simulink model "ImpedanceScanAndRecord_v2_for_RTLAB"  (R2020a)
settings: Solver=FixedStepDiscrete  StartTime=0.0  StopTime=30  RelTol=1e-3
InitFcn:
  | Ts = 50e-6;
libraries: dspsigops x16, powerlib x9
settings Model: Creator=anony  LastModifiedBy=anony

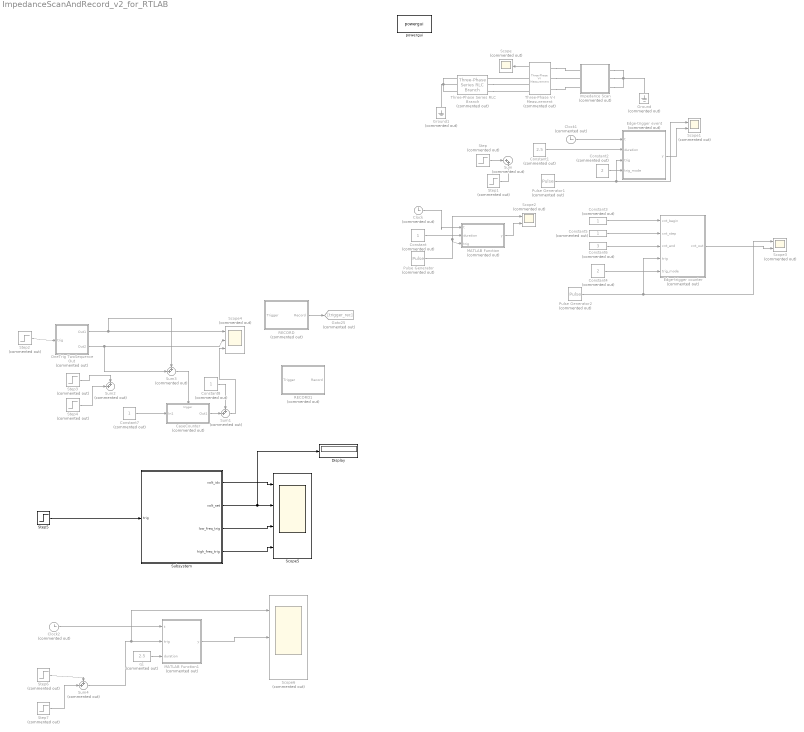
== system ImpedanceScanAndRecord_v2_for_RTLAB ==
  CaseCounter : Subsystem  Commented=on  TreatAsAtomicUnit=on
  Clock : Clock  Commented=on
  Clock1 : Clock  Commented=on
  Clock2 : Clock  Commented=on
  Constant{,3,5,7..8} (5 alike) : Constant  Commented=on
  Constant1 : Constant  Commented=on  Value=2.5
  Constant2 : Constant  Commented=on  Value=2
  Constant4 : Constant  Commented=on  Value=2
  Constant6 : Constant  Commented=on  Value=3
  Display : Display
  Edge-trigger counter : MATLAB Function  Commented=on  TreatAsAtomicUnit=on  SystemSampleTime=50e-6
  Edge-trigger event : MATLAB Function  Commented=on  TreatAsAtomicUnit=on  SystemSampleTime=50e-6
  Goto25 : Goto  Commented=on  GotoTag=trigger_rec
  Ground : powerlib/Elements/Ground  Commented=on  LConnTagsString=a
  Ground1 : powerlib/Elements/Ground  Commented=on  LConnTagsString=a
  Impedance Scan : Subsystem  Commented=on  mask{t_start=1, frequency=1, inject_duration=2, record_duration=1, stable_duration=1, amp_inject=690 * 0.1, t_Ts=Ts}
      mask prompts: t_start "启动时间 (s)"; frequency "待扫频率 (Hz)"; inject_duration "扰动时长 (s)"; record_duration "录波时长 (s)"; stable_duration "稳定时长 (s)"; amp_inject "扰动幅度 eg. 37e3 * 0.02"; t_Ts "Sample Ts"
  MATLAB Function : MATLAB Function  Commented=on  TreatAsAtomicUnit=on  SystemSampleTime=50e-6
  MATLAB Function1 : MATLAB Function  Commented=on  TreatAsAtomicUnit=on
  OneTrig TwoSequence Out : Subsystem  Commented=on  mask{var_delay=1, var_time_slot=0.5, var_dur_1=1, var_dur_2=2}
      mask prompts: var_delay "Time delay before start (s)"; var_time_slot "Time slot between step #1 and #2 (s)"; var_dur_1 "Step #1 duration (s)"; var_dur_2 "Step #2 duration (s)"
  Pulse Generator : DiscretePulseGenerator  Commented=on  PulseType=Time based  Period=1.2
  Pulse Generator1 : DiscretePulseGenerator  Commented=on  PulseType=Time based  Period=1  PulseWidth=10
  Pulse Generator2 : DiscretePulseGenerator  Commented=on  PulseType=Time based  Period=1  PulseWidth=10
  RECORD : Subsystem  Commented=on  mask{rec_time=15}
      mask prompts: rec_time "录波时长（s）"
  RECORD1 : Subsystem  Commented=on  mask{rec_time=15}
      mask prompts: rec_time "录波时长（s）"
  Scope : Scope  Commented=on
  Scope1 : Scope  Commented=on  NumInputPorts=2
  Scope2 : Scope  Commented=on  NumInputPorts=2
  Scope3 : Scope  Commented=on  NumInputPorts=2
  Scope4 : Scope  Commented=on  NumInputPorts=3
  Scope5 : Scope  NumInputPorts=4
  Scope6 : Scope  Commented=on  NumInputPorts=3
  Step : Step  Commented=on  SampleTime=0
  Step1 : Step  Commented=on  Time=1.5  After=-1  SampleTime=0
  Step2 : Step  Commented=on  SampleTime=0
  Step3 : Step  Commented=on  SampleTime=0
  Step4 : Step  Commented=on  Time=2  After=-1  SampleTime=0
  Step5 : Step  Time=0.1  SampleTime=0
  Step6 : Step  Commented=on  Time=0.1  SampleTime=0
  Step7 : Step  Commented=on  Time=0.2  After=-1  SampleTime=0
  Subsystem : Subsystem  mask{var_start_delay=2, var_low_dur=2.5, var_high_dur=2.26, voltage_vector=[0.95, 1.0, 1.05], var_myts=50e-4}
      mask prompts: var_start_delay "Delay before start (s)"; var_low_dur "Low frequency scan duration (s)"; var_high_dur "Hight frequency scan duration (s)"; voltage_vector "Voltage to be scanned. eg: [0.95, 1.0, 1.05]"; var_myts "Sample Time (s)"
  Sum : Sum  Commented=on  Inputs=|++
  Sum{1..4} (4 alike) : Sum  Commented=on  Inputs=++|
  Three-Phase Series RLC Branch : powerlib/Elements/Three-Phase Series RLC Branch  Commented=on  LConnTagsString=A|B|C  RConnTagsString=A|B|C  BranchType=R  Resistance=1  Inductance=1e-3  Capacitance=1e-6  Measurements=None
  Three-Phase V-I Measurement : powerlib/Measurements/Three-Phase V-I Measurement  Commented=on  VoltageMeasurement=phase-to-ground  SetLabelV=off  LabelV=Vabc  Vpu=off  VpuLL=off  CurrentMeasurement=yes  SetLabelI=off  LabelI=Iabc  Ipu=off  Pbase=100e6  Vbase=500e3  OutputType=Complex  PhasorSimulation=off  PSBequivalent=0
  powergui : powerlib/powergui  Priority=1  SimulationMode=Discrete  SampleTime=50e-6  frequency=60  Iterations=50  frequencyindice=0  Pbase=100e6  ErrMax=1e-4  UnitsV=kV  UnitsW=MW  buscounter=0  FunctionMessages=off  echomessages=off  EnableUseOfTLC=off  CurrentSourceSwitches=off  DisableSnubberDevices=off  DisableRonSwitches=off  DisableVfSwitches=off  DisplayEquations=off  AutomaticDiscreteSolvers=off  SolverType=Tustin/Backward Euler (TBE)  Interpol=off  ExternalGateDelay=off  methode=off  Ts=100  x0status=blocks  SPID=on  SwTol=0  HookPort=off  NonlinearTolerance=1e-4  nMaxIteration=100  ContinueOnMaxIteration=off  RestoreLinks=warning  ResistiveCurrentMeasurement=off  Frange=[0:2:500]  Ylog=off  Xlog=on  ShowGrid=off  save=off  variable=ZData  structure=0  ZoomFFT=off  StartTime=0.0  cycles=1  DisplayStyle=1  fundamental=60  FreqAxis=off  MaxFrequency=1000  frequencyindicesteady=1  RmsSteady=1  display=off
  q1 : Constant  Commented=on  Value=2.5
  wires:
  Three-Phase V-I Measurement/1 -> Scope/1
  Constant/1 -> MATLAB Function/2(duration)
  MATLAB Function/1(y) -> Scope2/2
  Pulse Generator/1 -> MATLAB Function/3(trig), Scope2/1
  Clock/1 -> MATLAB Function/1(t)
  Step/1 -> Sum/1
  Step1/1 -> Sum/2
  Constant1/1 -> Edge-trigger event/2(duration)
  Clock1/1 -> Edge-trigger event/1(t)
  Edge-trigger event/1(y) -> Scope1/2
  Constant2/1 -> Edge-trigger event/4(trig_mode)
  Pulse Generator1/1 -> Scope1/1, Edge-trigger event/3(trig)
  Pulse Generator2/1 -> Edge-trigger counter/4(trig), Scope3/1
  Constant4/1 -> Edge-trigger counter/5(trig_mode)
  Constant3/1 -> Edge-trigger counter/1(cnt_begin)
  Constant5/1 -> Edge-trigger counter/2(cnt_step)
  Constant6/1 -> Edge-trigger counter/3(cnt_end)
  Edge-trigger counter/1(cnt_out) -> Scope3/2
  q1/1 -> MATLAB Function1/3(duration)
  MATLAB Function1/1(y) -> Scope6/2
  Sum4/1 -> MATLAB Function1/2(trig), Scope6/1
  Step7/1 -> Sum4/2
  Step6/1 -> Sum4/1
  Clock2/1 -> MATLAB Function1/1(t)
  Subsystem/4(high_freq_trig) -> Scope5/4
  Subsystem/1(volt_idx) -> Scope5/1
  Subsystem/3(low_freq_trig) -> Scope5/3
  Subsystem/2(volt_set) -> Display/1, Scope5/2
  Step5/1 -> Subsystem/1(trig)
  Sum1/1 -> Scope4/3
  Sum3/1 -> CaseCounter/Trigger
  Step4/1 -> Sum2/2
  Step3/1 -> Sum2/1
  CaseCounter/1(Out1) -> Sum1/2
  Constant8/1 -> Sum1/1
  Constant7/1 -> CaseCounter/1(In1)
  Step2/1 -> OneTrig TwoSequence Out/1(trig)
  OneTrig TwoSequence Out/1(Out1) -> Scope4/1, Sum3/1
  OneTrig TwoSequence Out/2(Out2) -> Scope4/2, Sum3/2
  RECORD/1(Record) -> Goto25/1
  connections:
  Impedance Scan/LConn2 -- Impedance Scan/LConn1 -- Ground/LConn1 -- Impedance Scan/LConn3
  Ground1/LConn1 -- Three-Phase Series RLC Branch/LConn3 -- Three-Phase Series RLC Branch/LConn1 -- Three-Phase Series RLC Branch/LConn2
  Three-Phase V-I Measurement/LConn3 -- Impedance Scan/RConn3
  Three-Phase V-I Measurement/LConn2 -- Impedance Scan/RConn2
  Three-Phase V-I Measurement/LConn1 -- Impedance Scan/RConn1
  Three-Phase V-I Measurement/RConn1 -- Three-Phase Series RLC Branch/RConn1
  Three-Phase Series RLC Branch/RConn2 -- Three-Phase V-I Measurement/RConn2
  Three-Phase Series RLC Branch/RConn3 -- Three-Phase V-I Measurement/RConn3

== system ImpedanceScanAndRecord_v2_for_RTLAB/CaseCounter ==
  In1 : Inport
  Trigger : TriggerPort  TriggerType=falling  VariantControl=(inherit)
  Sum : Sum  Inputs=|++
  Unit Delay : UnitDelay  InitialCondition=1  SampleTime=-1  HasFrameUpgradeWarning=on
  Out1 : Outport
  wires:
  In1/1 -> Sum/1
  Sum/1 -> Unit Delay/1
  Unit Delay/1 -> Out1/1, Sum/2

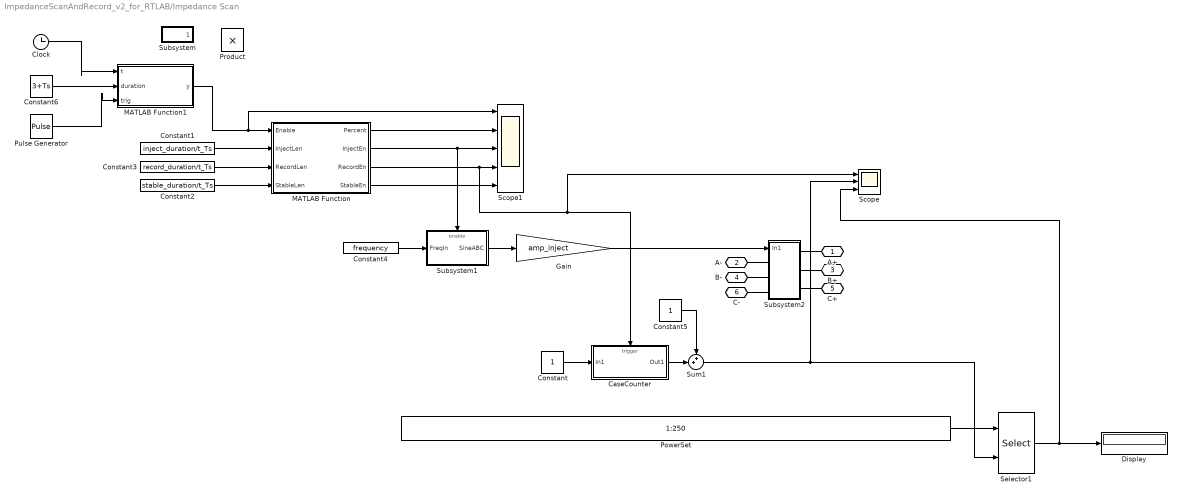
== system ImpedanceScanAndRecord_v2_for_RTLAB/Impedance Scan ==
  CaseCounter : Subsystem  TreatAsAtomicUnit=on
  Clock : Clock
  Constant : Constant
  Constant1 : Constant  Value=inject_duration/t_Ts
  Constant2 : Constant  Value=stable_duration/t_Ts
  Constant3 : Constant  Value=record_duration/t_Ts
  Constant4 : Constant  Value=frequency
  Constant5 : Constant
  Constant6 : Constant  Value=3+Ts
  Display : Display
  Gain : Gain  Gain=amp_inject
  MATLAB Function : MATLAB Function  TreatAsAtomicUnit=on  SystemSampleTime=t_Ts
  MATLAB Function1 : MATLAB Function  TreatAsAtomicUnit=on  SystemSampleTime=50e-6
  PowerSet : Constant  Value=1:250
  Product : Product
  Pulse Generator : DiscretePulseGenerator  PulseType=Time based  Period=3*1.03
  Scope : Scope  NumInputPorts=3
  Scope1 : Scope  NumInputPorts=5
  Selector1 : Selector  InputPortWidth=250  IndexOptions=Index vector (port)  Indices=[1 3]  OutputSizes=1
  Subsystem : Subsystem  mask{t_start=t_start, t_duration=inject_duration + stable_duration}
      mask prompts: t_start "Start Time"; t_duration "Duration"
  Subsystem1 : Subsystem
  Subsystem2 : Subsystem
  Sum1 : Sum  Inputs=++|
  A+ : PMIOPort  Side=Right
  A- : PMIOPort  Port=2  Side=Left
  B+ : PMIOPort  Port=3  Side=Right
  B- : PMIOPort  Port=4  Side=Left
  C+ : PMIOPort  Port=5  Side=Right
  C- : PMIOPort  Port=6  Side=Left
  wires:
  MATLAB Function/1(Percent) -> Scope1/2
  Constant1/1 -> MATLAB Function/2(InjectLen)
  Constant2/1 -> MATLAB Function/4(StableLen)
  Constant3/1 -> MATLAB Function/3(RecordLen)
  MATLAB Function/2(InjectEn) -> Subsystem1/Enable, Scope1/3
  MATLAB Function/4(StableEn) -> Scope1/5
  Constant4/1 -> Subsystem1/1(FreqIn)
  Subsystem1/1(SineABC) -> Gain/1
  Gain/1 -> Subsystem2/1(In1)
  Sum1/1 -> Selector1/2, Scope/2
  Constant/1 -> CaseCounter/1(In1)
  Constant5/1 -> Sum1/1
  CaseCounter/1(Out1) -> Sum1/2
  MATLAB Function/3(RecordEn) -> Scope/1, CaseCounter/Trigger, Scope1/4
  Selector1/1 -> Scope/3, Display/1
  PowerSet/1 -> Selector1/1
  Constant6/1 -> MATLAB Function1/2(duration)
  Pulse Generator/1 -> MATLAB Function1/3(trig)
  Clock/1 -> MATLAB Function1/1(t)
  MATLAB Function1/1(y) -> Scope1/1, MATLAB Function/1(Enable)
  connections:
  Subsystem2/RConn3 -- C+/RConn1
  Subsystem2/LConn1 -- A-/RConn1
  Subsystem2/LConn2 -- B-/RConn1
  Subsystem2/LConn3 -- C-/RConn1
  Subsystem2/RConn1 -- A+/RConn1
  Subsystem2/RConn2 -- B+/RConn1

== system ImpedanceScanAndRecord_v2_for_RTLAB/OneTrig TwoSequence Out ==
  trig : Inport
  Constant1 : Constant  Value=var_dur_1
  Constant2 : Constant  Value=var_delay
  Constant3 : Constant  Value=var_delay + var_dur_1 + var_time_slot
  Constant4 : Constant  Value=var_dur_2
  StepTrig#1 : Subsystem
  StepTrig#2 : Subsystem
  Out1 : Outport
  Out2 : Outport  Port=2
  wires:
  Constant4/1 -> StepTrig#2/3(Duration)
  Constant3/1 -> StepTrig#2/2(Delay)
  Constant1/1 -> StepTrig#1/3(Duration)
  StepTrig#1/1(Out) -> Out1/1
  StepTrig#2/1(Out) -> Out2/1
  trig/1 -> StepTrig#1/1(Trigger), StepTrig#2/1(Trigger)
  Constant2/1 -> StepTrig#1/2(Delay)

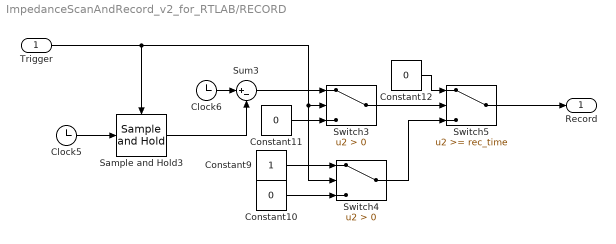
== system ImpedanceScanAndRecord_v2_for_RTLAB/RECORD ==
  Trigger : Inport
  Clock5 : Clock
  Clock6 : Clock
      settings: DisableCoverage=on
  Constant10 : Constant  Value=0
  Constant11 : Constant  Value=0
  Constant12 : Constant  Value=0
  Constant9 : Constant
  Sample and Hold3 : dspsigops/Sample and Hold  trig=Rising edge  initCond=0  latchinput=off
  Sum3 : Sum  DisableCoverage=on  Inputs=|+-  InputSameDT=on  SaturateOnIntegerOverflow=on  OutDataTypeStr=Inherit: Same as first input
  Switch3 : Switch  Criteria=u2 > Threshold
  Switch4 : Switch  Criteria=u2 > Threshold
  Switch5 : Switch  Threshold=rec_time
  Record : Outport
  wires:
  Constant10/1 -> Switch4/3
  Constant12/1 -> Switch5/1
  Sample and Hold3/1 -> Sum3/2
  Clock6/1 -> Sum3/1
  Switch4/1 -> Switch5/3
  Constant11/1 -> Switch3/3
  Constant9/1 -> Switch4/1
  Sum3/1 -> Switch3/1
  Clock5/1 -> Sample and Hold3/1
  Switch3/1 -> Switch5/2
  Trigger/1 -> Switch4/2, Switch3/2, Sample and Hold3/Trigger
  Switch5/1 -> Record/1

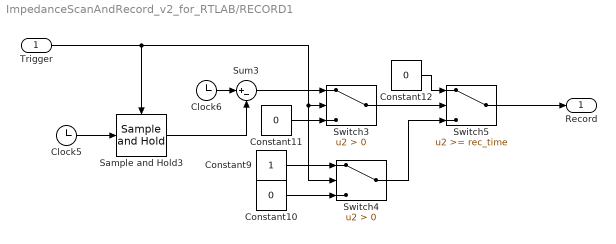
== system ImpedanceScanAndRecord_v2_for_RTLAB/RECORD1 ==
  Trigger : Inport
  Clock5 : Clock
  Clock6 : Clock
      settings: DisableCoverage=on
  Constant10 : Constant  Value=0
  Constant11 : Constant  Value=0
  Constant12 : Constant  Value=0
  Constant9 : Constant
  Sample and Hold3 : dspsigops/Sample and Hold  trig=Rising edge  initCond=0  latchinput=off
  Sum3 : Sum  DisableCoverage=on  Inputs=|+-  InputSameDT=on  SaturateOnIntegerOverflow=on  OutDataTypeStr=Inherit: Same as first input
  Switch3 : Switch  Criteria=u2 > Threshold
  Switch4 : Switch  Criteria=u2 > Threshold
  Switch5 : Switch  Threshold=rec_time
  Record : Outport
  wires:
  Switch5/1 -> Record/1
  Trigger/1 -> Sample and Hold3/Trigger, Switch3/2, Switch4/2
  Switch3/1 -> Switch5/2
  Clock5/1 -> Sample and Hold3/1
  Sum3/1 -> Switch3/1
  Constant9/1 -> Switch4/1
  Constant11/1 -> Switch3/3
  Switch4/1 -> Switch5/3
  Clock6/1 -> Sum3/1
  Sample and Hold3/1 -> Sum3/2
  Constant12/1 -> Switch5/1
  Constant10/1 -> Switch4/3

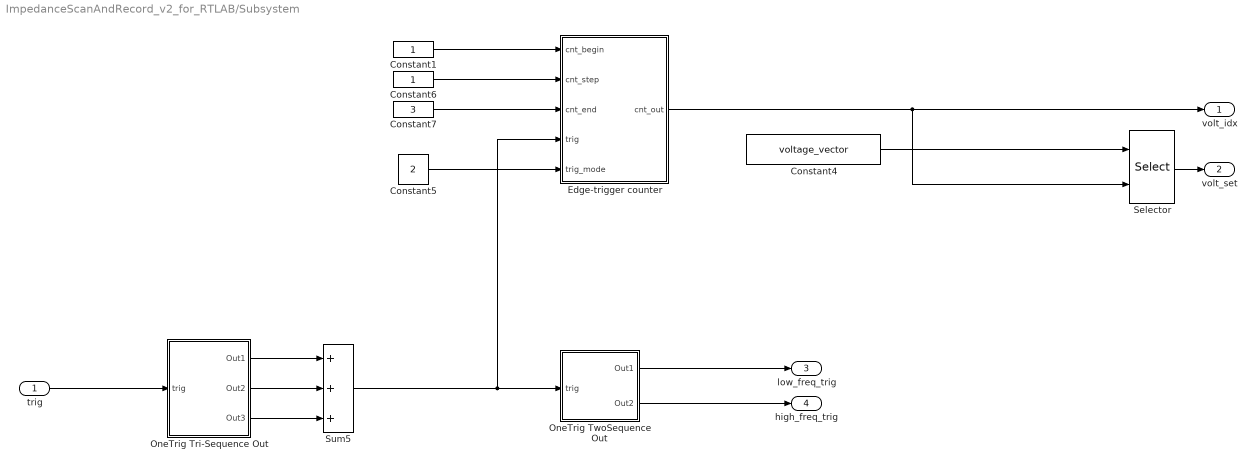
== system ImpedanceScanAndRecord_v2_for_RTLAB/Subsystem ==
  trig : Inport
  Constant1 : Constant
  Constant4 : Constant  Value=voltage_vector
  Constant5 : Constant  Value=2
  Constant6 : Constant
  Constant7 : Constant  Value=3
  Edge-trigger counter : MATLAB Function  TreatAsAtomicUnit=on  SystemSampleTime=50e-6
  OneTrig Tri-Sequence Out : Subsystem  mask{var_delay=0.1, var_time_slot=0.2, var_dur_1=var_low_dur + var_high_dur + 4, var_dur_2=var_low_dur + var_high_dur + 4, var_dur_3=var_low_dur + var_high_dur + 4}
      mask prompts: var_delay "Time delay before start (s)"; var_time_slot "Time slot between steps (s)"; var_dur_1 "Step #1 duration (s)"; var_dur_2 "Step #2 duration (s)"; var_dur_3 "Step #3 duration (s)"
  OneTrig TwoSequence Out : Subsystem  mask{var_delay=0.5, var_time_slot=1, var_dur_1=var_low_dur+1, var_dur_2=var_high_dur+1}
      mask prompts: var_delay "Time delay before start (s)"; var_time_slot "Time slot between step #1 and #2 (s)"; var_dur_1 "Step #1 duration (s)"; var_dur_2 "Step #2 duration (s)"
  Selector : Selector  InputPortWidth=length(voltage_vector)  SampleTime=var_myts  IndexOptions=Index vector (port)  Indices=[1 3]  OutputSizes=1
  Sum5 : Sum  Inputs=+++  SampleTime=var_myts
  volt_idx : Outport
  volt_set : Outport  Port=2
  low_freq_trig : Outport  Port=3
  high_freq_trig : Outport  Port=4
  wires:
  OneTrig TwoSequence Out/2(Out2) -> high_freq_trig/1
  OneTrig TwoSequence Out/1(Out1) -> low_freq_trig/1
  Edge-trigger counter/1(cnt_out) -> Selector/2, volt_idx/1
  Constant4/1 -> Selector/1
  Selector/1 -> volt_set/1
  OneTrig Tri-Sequence Out/1(Out1) -> Sum5/1
  trig/1 -> OneTrig Tri-Sequence Out/1(trig)
  OneTrig Tri-Sequence Out/2(Out2) -> Sum5/2
  OneTrig Tri-Sequence Out/3(Out3) -> Sum5/3
  Constant6/1 -> Edge-trigger counter/2(cnt_step)
  Sum5/1 -> Edge-trigger counter/4(trig), OneTrig TwoSequence Out/1(trig)
  Constant5/1 -> Edge-trigger counter/5(trig_mode)
  Constant7/1 -> Edge-trigger counter/3(cnt_end)
  Constant1/1 -> Edge-trigger counter/1(cnt_begin)

== system ImpedanceScanAndRecord_v2_for_RTLAB/Impedance Scan/CaseCounter ==
  In1 : Inport
  Trigger : TriggerPort  TriggerType=falling  VariantControl=(inherit)
  Sum : Sum  Inputs=|++
  Unit Delay : UnitDelay  InitialCondition=1  SampleTime=-1  HasFrameUpgradeWarning=on
  Out1 : Outport
  wires:
  In1/1 -> Sum/1
  Sum/1 -> Unit Delay/1
  Unit Delay/1 -> Out1/1, Sum/2

== system ImpedanceScanAndRecord_v2_for_RTLAB/Impedance Scan/Subsystem ==
  Step : Step  Time=t_start  SampleTime=t_Ts
  Step1 : Step  Time=t_start+t_duration  After=-1  SampleTime=t_Ts
  Sum : Sum  Inputs=|++
  EnOut : Outport
  wires:
  Step1/1 -> Sum/2
  Step/1 -> Sum/1
  Sum/1 -> EnOut/1

== system ImpedanceScanAndRecord_v2_for_RTLAB/Impedance Scan/Subsystem1 ==
  FreqIn : Inport
  Enable : EnablePort
  Clock : Clock
  Fcn : Fcn  Expr=sin(2*pi*u(1)*u(2))
  Fcn1 : Fcn  Expr=sin(2*pi*u(1)*u(2) - 2*pi/3)
  Fcn2 : Fcn  Expr=sin(2*pi*u(1)*u(2) + 2*pi/3)
  Mux : Mux  Inputs=3
  Mux1 : Mux  Inputs=2
  SineABC : Outport
  wires:
  Clock/1 -> Mux1/2
  FreqIn/1 -> Mux1/1
  Mux1/1 -> Fcn1/1, Fcn/1, Fcn2/1
  Mux/1 -> SineABC/1
  Fcn2/1 -> Mux/3
  Fcn/1 -> Mux/1
  Fcn1/1 -> Mux/2

== system ImpedanceScanAndRecord_v2_for_RTLAB/Impedance Scan/Subsystem2 ==
  In1 : Inport
  Controlled Voltage Source : powerlib/Electrical Sources/Controlled Voltage Source  Initialize=on  Source_Type=AC  Amplitude=0  Phase=0  Frequency=0  Measurements=None
  Controlled Voltage Source1 : powerlib/Electrical Sources/Controlled Voltage Source  Initialize=on  Source_Type=AC  Amplitude=0  Phase=0  Frequency=0  Measurements=None
  Controlled Voltage Source2 : powerlib/Electrical Sources/Controlled Voltage Source  Initialize=on  Source_Type=AC  Amplitude=0  Phase=0  Frequency=0  Measurements=None
  Demux : Demux  Outputs=3
  Vabc/Iabc to Record : powerlib/Measurements/Three-Phase V-I Measurement  VoltageMeasurement=phase-to-ground  SetLabelV=on  LabelV=ScanVabc  Vpu=off  VpuLL=off  CurrentMeasurement=yes  SetLabelI=on  LabelI=ScanIabc  Ipu=off  Pbase=100e6  Vbase=500e3  OutputType=Complex  PhasorSimulation=off  PSBequivalent=0
  A- : PMIOPort  Side=Left
  A+ : PMIOPort  Port=2  Side=Right
  B+ : PMIOPort  Port=3  Side=Right
  B- : PMIOPort  Port=4  Side=Left
  C+ : PMIOPort  Port=5  Side=Right
  C- : PMIOPort  Port=6  Side=Left
  wires:
  In1/1 -> Demux/1
  Demux/1 -> Controlled Voltage Source/1
  Demux/2 -> Controlled Voltage Source1/1
  Demux/3 -> Controlled Voltage Source2/1
  connections:
  Controlled Voltage Source2/LConn1 -- C-/RConn1
  Vabc/Iabc to Record/RConn2 -- B+/RConn1
  Controlled Voltage Source1/LConn1 -- B-/RConn1
  Controlled Voltage Source/LConn1 -- A-/RConn1
  Vabc/Iabc to Record/RConn3 -- C+/RConn1
  Controlled Voltage Source2/RConn1 -- Vabc/Iabc to Record/LConn3
  Controlled Voltage Source1/RConn1 -- Vabc/Iabc to Record/LConn2
  Controlled Voltage Source/RConn1 -- Vabc/Iabc to Record/LConn1
  Vabc/Iabc to Record/RConn1 -- A+/RConn1

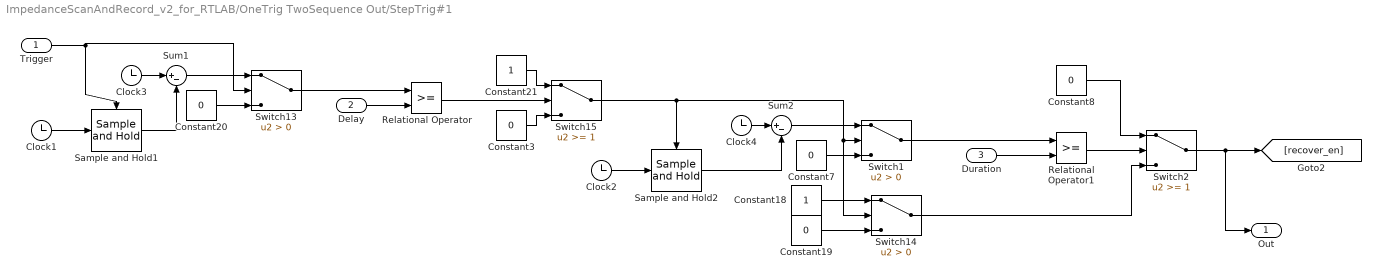
== system ImpedanceScanAndRecord_v2_for_RTLAB/OneTrig TwoSequence Out/StepTrig#1 ==
  Trigger : Inport
  Delay : Inport  Port=2
  Duration : Inport  Port=3
  Clock{1..4} (4 alike) : Clock
      Clock3 settings: DisableCoverage=on
      Clock4 settings: DisableCoverage=on
  Constant18 : Constant
  Constant{3,7..8,19..20} (5 alike) : Constant  Value=0
  Constant21 : Constant
  Relational Operator : RelationalOperator  OutDataTypeStr=boolean  RndMeth=Nearest
  Relational Operator1 : RelationalOperator  OutDataTypeStr=boolean  RndMeth=Nearest
  Sample and Hold1 : dspsigops/Sample and Hold  trig=Rising edge  initCond=0  latchinput=off
  Sample and Hold2 : dspsigops/Sample and Hold  trig=Rising edge  initCond=0  latchinput=off
  Sum1 : Sum  DisableCoverage=on  Inputs=|+-  InputSameDT=on  SaturateOnIntegerOverflow=on  OutDataTypeStr=Inherit: Same as first input
  Sum2 : Sum  DisableCoverage=on  Inputs=|+-  InputSameDT=on  SaturateOnIntegerOverflow=on  OutDataTypeStr=Inherit: Same as first input
  Switch1 : Switch  Criteria=u2 > Threshold
  Switch13 : Switch  Criteria=u2 > Threshold
  Switch14 : Switch  Criteria=u2 > Threshold
  Switch15 : Switch  Threshold=1
  Switch2 : Switch  Threshold=1
  Out : Outport
  wires:
  Duration/1 -> Relational Operator1/2
  Switch1/1 -> Relational Operator1/1
  Relational Operator1/1 -> Switch2/2
  Relational Operator/1 -> Switch15/2
  Delay/1 -> Relational Operator/2
  Switch13/1 -> Relational Operator/1
  Clock2/1 -> Sample and Hold2/1
  Sum2/1 -> Switch1/1
  Constant18/1 -> Switch14/1
  Sample and Hold2/1 -> Sum2/2
  Constant8/1 -> Switch2/1
  Clock4/1 -> Sum2/1
  Constant7/1 -> Switch1/3
  Switch14/1 -> Switch2/3
  Constant19/1 -> Switch14/3
  Sample and Hold1/1 -> Sum1/2
  Clock1/1 -> Sample and Hold1/1
  Constant20/1 -> Switch13/3
  Sum1/1 -> Switch13/1
  Constant21/1 -> Switch15/1
  Constant3/1 -> Switch15/3
  Clock3/1 -> Sum1/1
  Switch15/1 -> Sample and Hold2/Trigger, Switch14/2, Switch1/2
  Trigger/1 -> Switch13/2, Sample and Hold1/Trigger
  Switch2/1 -> Out/1, [recover_en]

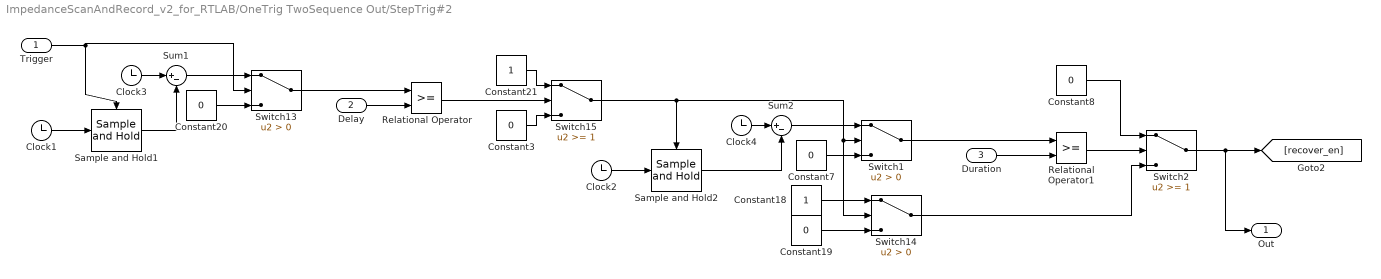
== system ImpedanceScanAndRecord_v2_for_RTLAB/OneTrig TwoSequence Out/StepTrig#2 ==
  Trigger : Inport
  Delay : Inport  Port=2
  Duration : Inport  Port=3
  Clock{1..4} (4 alike) : Clock
      Clock3 settings: DisableCoverage=on
      Clock4 settings: DisableCoverage=on
  Constant18 : Constant
  Constant{3,7..8,19..20} (5 alike) : Constant  Value=0
  Constant21 : Constant
  Relational Operator : RelationalOperator  OutDataTypeStr=boolean  RndMeth=Nearest
  Relational Operator1 : RelationalOperator  OutDataTypeStr=boolean  RndMeth=Nearest
  Sample and Hold1 : dspsigops/Sample and Hold  trig=Rising edge  initCond=0  latchinput=off
  Sample and Hold2 : dspsigops/Sample and Hold  trig=Rising edge  initCond=0  latchinput=off
  Sum1 : Sum  DisableCoverage=on  Inputs=|+-  InputSameDT=on  SaturateOnIntegerOverflow=on  OutDataTypeStr=Inherit: Same as first input
  Sum2 : Sum  DisableCoverage=on  Inputs=|+-  InputSameDT=on  SaturateOnIntegerOverflow=on  OutDataTypeStr=Inherit: Same as first input
  Switch1 : Switch  Criteria=u2 > Threshold
  Switch13 : Switch  Criteria=u2 > Threshold
  Switch14 : Switch  Criteria=u2 > Threshold
  Switch15 : Switch  Threshold=1
  Switch2 : Switch  Threshold=1
  Out : Outport
  wires:
  Switch2/1 -> [recover_en], Out/1
  Trigger/1 -> Sample and Hold1/Trigger, Switch13/2
  Switch15/1 -> Switch1/2, Switch14/2, Sample and Hold2/Trigger
  Clock3/1 -> Sum1/1
  Constant3/1 -> Switch15/3
  Constant21/1 -> Switch15/1
  Sum1/1 -> Switch13/1
  Constant20/1 -> Switch13/3
  Clock1/1 -> Sample and Hold1/1
  Sample and Hold1/1 -> Sum1/2
  Constant19/1 -> Switch14/3
  Switch14/1 -> Switch2/3
  Constant7/1 -> Switch1/3
  Clock4/1 -> Sum2/1
  Constant8/1 -> Switch2/1
  Sample and Hold2/1 -> Sum2/2
  Constant18/1 -> Switch14/1
  Sum2/1 -> Switch1/1
  Clock2/1 -> Sample and Hold2/1
  Switch13/1 -> Relational Operator/1
  Delay/1 -> Relational Operator/2
  Relational Operator/1 -> Switch15/2
  Relational Operator1/1 -> Switch2/2
  Switch1/1 -> Relational Operator1/1
  Duration/1 -> Relational Operator1/2

== system ImpedanceScanAndRecord_v2_for_RTLAB/Subsystem/OneTrig Tri-Sequence Out ==
  trig : Inport
  Constant1 : Constant  Value=var_dur_1
  Constant2 : Constant  Value=var_delay
  Constant3 : Constant  Value=var_delay + var_dur_1 + var_time_slot
  Constant4 : Constant  Value=var_dur_2
  Constant5 : Constant  Value=var_delay + var_dur_1 + var_time_slot + var_dur_2 + var_time_slot
  Constant6 : Constant  Value=var_dur_2
  StepTrig#1 : Subsystem
  StepTrig#2 : Subsystem
  StepTrig#3 : Subsystem
  Out1 : Outport
  Out2 : Outport  Port=2
  Out3 : Outport  Port=3
  wires:
  StepTrig#3/1(Out) -> Out3/1
  trig/1 -> StepTrig#2/1(Trigger), StepTrig#3/1(Trigger), StepTrig#1/1(Trigger)
  Constant5/1 -> StepTrig#3/2(Delay)
  Constant6/1 -> StepTrig#3/3(Duration)
  Constant2/1 -> StepTrig#1/2(Delay)
  StepTrig#2/1(Out) -> Out2/1
  StepTrig#1/1(Out) -> Out1/1
  Constant1/1 -> StepTrig#1/3(Duration)
  Constant3/1 -> StepTrig#2/2(Delay)
  Constant4/1 -> StepTrig#2/3(Duration)

== system ImpedanceScanAndRecord_v2_for_RTLAB/Subsystem/OneTrig TwoSequence Out ==
  trig : Inport
  Constant1 : Constant  Value=var_dur_1
  Constant2 : Constant  Value=var_delay
  Constant3 : Constant  Value=var_delay + var_dur_1 + var_time_slot
  Constant4 : Constant  Value=var_dur_2
  StepTrig#1 : Subsystem
  StepTrig#2 : Subsystem
  Out1 : Outport
  Out2 : Outport  Port=2
  wires:
  Constant4/1 -> StepTrig#2/3(Duration)
  Constant3/1 -> StepTrig#2/2(Delay)
  Constant1/1 -> StepTrig#1/3(Duration)
  StepTrig#1/1(Out) -> Out1/1
  StepTrig#2/1(Out) -> Out2/1
  trig/1 -> StepTrig#1/1(Trigger), StepTrig#2/1(Trigger)
  Constant2/1 -> StepTrig#1/2(Delay)

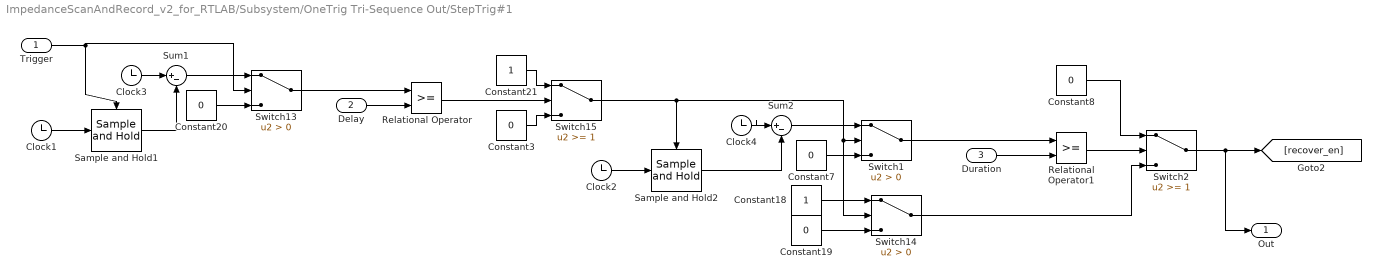
== system ImpedanceScanAndRecord_v2_for_RTLAB/Subsystem/OneTrig Tri-Sequence Out/StepTrig#1 ==
  Trigger : Inport
  Delay : Inport  Port=2
  Duration : Inport  Port=3
  Clock{1..4} (4 alike) : Clock
      Clock3 settings: DisableCoverage=on
      Clock4 settings: DisableCoverage=on
  Constant18 : Constant
  Constant{3,7..8,19..20} (5 alike) : Constant  Value=0
  Constant21 : Constant
  Relational Operator : RelationalOperator  OutDataTypeStr=boolean  RndMeth=Nearest
  Relational Operator1 : RelationalOperator  OutDataTypeStr=boolean  RndMeth=Nearest
  Sample and Hold1 : dspsigops/Sample and Hold  trig=Rising edge  initCond=0  latchinput=off
  Sample and Hold2 : dspsigops/Sample and Hold  trig=Rising edge  initCond=0  latchinput=off
  Sum1 : Sum  DisableCoverage=on  Inputs=|+-  InputSameDT=on  SaturateOnIntegerOverflow=on  OutDataTypeStr=Inherit: Same as first input
  Sum2 : Sum  DisableCoverage=on  Inputs=|+-  InputSameDT=on  SaturateOnIntegerOverflow=on  OutDataTypeStr=Inherit: Same as first input
  Switch1 : Switch  Criteria=u2 > Threshold  SampleTime=var_myts
  Switch13 : Switch  Criteria=u2 > Threshold  SampleTime=var_myts
  Switch14 : Switch  Criteria=u2 > Threshold  SampleTime=var_myts
  Switch15 : Switch  Threshold=1  SampleTime=var_myts
  Switch2 : Switch  Threshold=1  SampleTime=var_myts
  Out : Outport
  wires:
  Switch2/1 -> [recover_en], Out/1
  Trigger/1 -> Sample and Hold1/Trigger, Switch13/2
  Switch15/1 -> Switch1/2, Switch14/2, Sample and Hold2/Trigger
  Clock3/1 -> Sum1/1
  Constant3/1 -> Switch15/3
  Constant21/1 -> Switch15/1
  Sum1/1 -> Switch13/1
  Constant20/1 -> Switch13/3
  Clock1/1 -> Sample and Hold1/1
  Sample and Hold1/1 -> Sum1/2
  Constant19/1 -> Switch14/3
  Switch14/1 -> Switch2/3
  Constant7/1 -> Switch1/3
  Clock4/1 -> Sum2/1
  Constant8/1 -> Switch2/1
  Sample and Hold2/1 -> Sum2/2
  Constant18/1 -> Switch14/1
  Sum2/1 -> Switch1/1
  Clock2/1 -> Sample and Hold2/1
  Switch13/1 -> Relational Operator/1
  Delay/1 -> Relational Operator/2
  Relational Operator/1 -> Switch15/2
  Relational Operator1/1 -> Switch2/2
  Switch1/1 -> Relational Operator1/1
  Duration/1 -> Relational Operator1/2

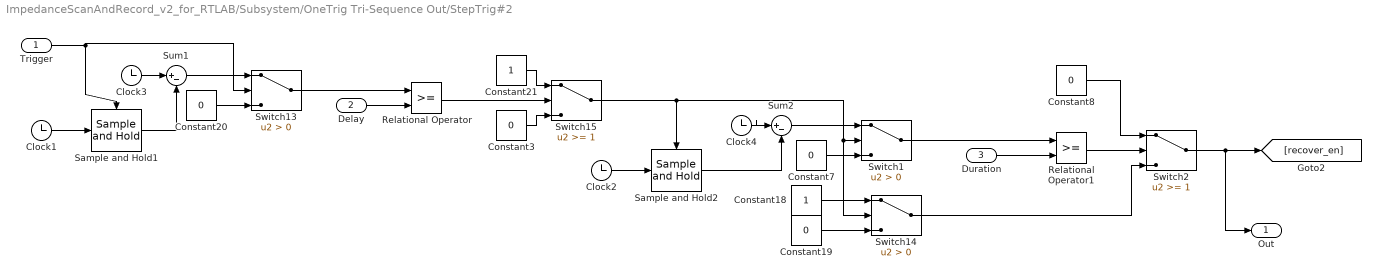
== system ImpedanceScanAndRecord_v2_for_RTLAB/Subsystem/OneTrig Tri-Sequence Out/StepTrig#2 ==
  Trigger : Inport
  Delay : Inport  Port=2
  Duration : Inport  Port=3
  Clock{1..4} (4 alike) : Clock
      Clock3 settings: DisableCoverage=on
      Clock4 settings: DisableCoverage=on
  Constant18 : Constant
  Constant{3,7..8,19..20} (5 alike) : Constant  Value=0
  Constant21 : Constant
  Relational Operator : RelationalOperator  OutDataTypeStr=boolean  RndMeth=Nearest
  Relational Operator1 : RelationalOperator  OutDataTypeStr=boolean  RndMeth=Nearest
  Sample and Hold1 : dspsigops/Sample and Hold  trig=Rising edge  initCond=0  latchinput=off
  Sample and Hold2 : dspsigops/Sample and Hold  trig=Rising edge  initCond=0  latchinput=off
  Sum1 : Sum  DisableCoverage=on  Inputs=|+-  InputSameDT=on  SaturateOnIntegerOverflow=on  OutDataTypeStr=Inherit: Same as first input
  Sum2 : Sum  DisableCoverage=on  Inputs=|+-  InputSameDT=on  SaturateOnIntegerOverflow=on  OutDataTypeStr=Inherit: Same as first input
  Switch1 : Switch  Criteria=u2 > Threshold  SampleTime=var_myts
  Switch13 : Switch  Criteria=u2 > Threshold  SampleTime=var_myts
  Switch14 : Switch  Criteria=u2 > Threshold  SampleTime=var_myts
  Switch15 : Switch  Threshold=1  SampleTime=var_myts
  Switch2 : Switch  Threshold=1  SampleTime=var_myts
  Out : Outport
  wires:
  Duration/1 -> Relational Operator1/2
  Switch1/1 -> Relational Operator1/1
  Relational Operator1/1 -> Switch2/2
  Relational Operator/1 -> Switch15/2
  Delay/1 -> Relational Operator/2
  Switch13/1 -> Relational Operator/1
  Clock2/1 -> Sample and Hold2/1
  Sum2/1 -> Switch1/1
  Constant18/1 -> Switch14/1
  Sample and Hold2/1 -> Sum2/2
  Constant8/1 -> Switch2/1
  Clock4/1 -> Sum2/1
  Constant7/1 -> Switch1/3
  Switch14/1 -> Switch2/3
  Constant19/1 -> Switch14/3
  Sample and Hold1/1 -> Sum1/2
  Clock1/1 -> Sample and Hold1/1
  Constant20/1 -> Switch13/3
  Sum1/1 -> Switch13/1
  Constant21/1 -> Switch15/1
  Constant3/1 -> Switch15/3
  Clock3/1 -> Sum1/1
  Switch15/1 -> Sample and Hold2/Trigger, Switch14/2, Switch1/2
  Trigger/1 -> Switch13/2, Sample and Hold1/Trigger
  Switch2/1 -> Out/1, [recover_en]

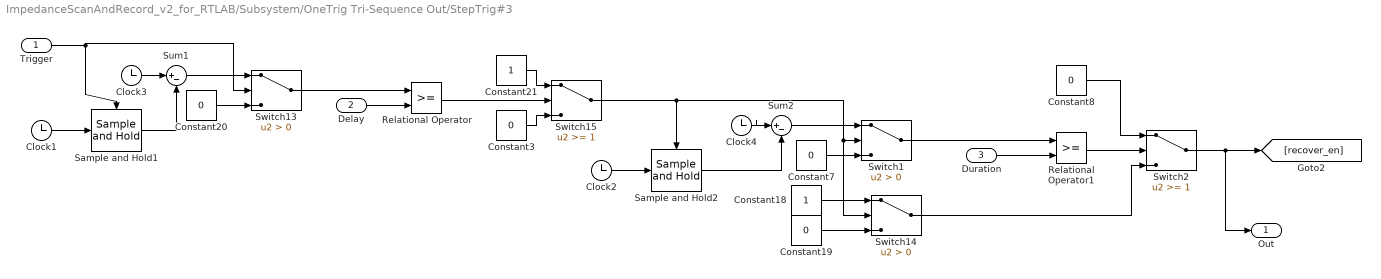
== system ImpedanceScanAndRecord_v2_for_RTLAB/Subsystem/OneTrig Tri-Sequence Out/StepTrig#3 ==
  Trigger : Inport
  Delay : Inport  Port=2
  Duration : Inport  Port=3
  Clock{1..4} (4 alike) : Clock
      Clock3 settings: DisableCoverage=on
      Clock4 settings: DisableCoverage=on
  Constant18 : Constant
  Constant{3,7..8,19..20} (5 alike) : Constant  Value=0
  Constant21 : Constant
  Relational Operator : RelationalOperator  OutDataTypeStr=boolean  RndMeth=Nearest
  Relational Operator1 : RelationalOperator  OutDataTypeStr=boolean  RndMeth=Nearest
  Sample and Hold1 : dspsigops/Sample and Hold  trig=Rising edge  initCond=0  latchinput=off
  Sample and Hold2 : dspsigops/Sample and Hold  trig=Rising edge  initCond=0  latchinput=off
  Sum1 : Sum  DisableCoverage=on  Inputs=|+-  InputSameDT=on  SaturateOnIntegerOverflow=on  OutDataTypeStr=Inherit: Same as first input
  Sum2 : Sum  DisableCoverage=on  Inputs=|+-  InputSameDT=on  SaturateOnIntegerOverflow=on  OutDataTypeStr=Inherit: Same as first input
  Switch1 : Switch  Criteria=u2 > Threshold  SampleTime=var_myts
  Switch13 : Switch  Criteria=u2 > Threshold  SampleTime=var_myts
  Switch14 : Switch  Criteria=u2 > Threshold  SampleTime=var_myts
  Switch15 : Switch  Threshold=1  SampleTime=var_myts
  Switch2 : Switch  Threshold=1  SampleTime=var_myts
  Out : Outport
  wires:
  Switch2/1 -> [recover_en], Out/1
  Trigger/1 -> Sample and Hold1/Trigger, Switch13/2
  Switch15/1 -> Switch1/2, Switch14/2, Sample and Hold2/Trigger
  Clock3/1 -> Sum1/1
  Constant3/1 -> Switch15/3
  Constant21/1 -> Switch15/1
  Sum1/1 -> Switch13/1
  Constant20/1 -> Switch13/3
  Clock1/1 -> Sample and Hold1/1
  Sample and Hold1/1 -> Sum1/2
  Constant19/1 -> Switch14/3
  Switch14/1 -> Switch2/3
  Constant7/1 -> Switch1/3
  Clock4/1 -> Sum2/1
  Constant8/1 -> Switch2/1
  Sample and Hold2/1 -> Sum2/2
  Constant18/1 -> Switch14/1
  Sum2/1 -> Switch1/1
  Clock2/1 -> Sample and Hold2/1
  Switch13/1 -> Relational Operator/1
  Delay/1 -> Relational Operator/2
  Relational Operator/1 -> Switch15/2
  Relational Operator1/1 -> Switch2/2
  Switch1/1 -> Relational Operator1/1
  Duration/1 -> Relational Operator1/2

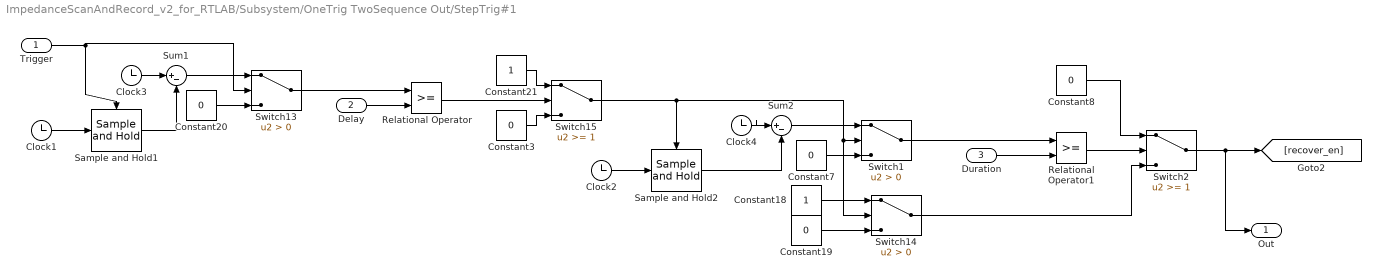
== system ImpedanceScanAndRecord_v2_for_RTLAB/Subsystem/OneTrig TwoSequence Out/StepTrig#1 ==
  Trigger : Inport
  Delay : Inport  Port=2
  Duration : Inport  Port=3
  Clock{1..4} (4 alike) : Clock
      Clock3 settings: DisableCoverage=on
      Clock4 settings: DisableCoverage=on
  Constant18 : Constant
  Constant{3,7..8,19..20} (5 alike) : Constant  Value=0
  Constant21 : Constant
  Relational Operator : RelationalOperator  OutDataTypeStr=boolean  RndMeth=Nearest
  Relational Operator1 : RelationalOperator  OutDataTypeStr=boolean  RndMeth=Nearest
  Sample and Hold1 : dspsigops/Sample and Hold  trig=Rising edge  initCond=0  latchinput=off
  Sample and Hold2 : dspsigops/Sample and Hold  trig=Rising edge  initCond=0  latchinput=off
  Sum1 : Sum  DisableCoverage=on  Inputs=|+-  InputSameDT=on  SaturateOnIntegerOverflow=on  OutDataTypeStr=Inherit: Same as first input
  Sum2 : Sum  DisableCoverage=on  Inputs=|+-  InputSameDT=on  SaturateOnIntegerOverflow=on  OutDataTypeStr=Inherit: Same as first input
  Switch1 : Switch  Criteria=u2 > Threshold  SampleTime=var_myts
  Switch13 : Switch  Criteria=u2 > Threshold  SampleTime=var_myts
  Switch14 : Switch  Criteria=u2 > Threshold  SampleTime=var_myts
  Switch15 : Switch  Threshold=1  SampleTime=var_myts
  Switch2 : Switch  Threshold=1  SampleTime=var_myts
  Out : Outport
  wires:
  Duration/1 -> Relational Operator1/2
  Switch1/1 -> Relational Operator1/1
  Relational Operator1/1 -> Switch2/2
  Relational Operator/1 -> Switch15/2
  Delay/1 -> Relational Operator/2
  Switch13/1 -> Relational Operator/1
  Clock2/1 -> Sample and Hold2/1
  Sum2/1 -> Switch1/1
  Constant18/1 -> Switch14/1
  Sample and Hold2/1 -> Sum2/2
  Constant8/1 -> Switch2/1
  Clock4/1 -> Sum2/1
  Constant7/1 -> Switch1/3
  Switch14/1 -> Switch2/3
  Constant19/1 -> Switch14/3
  Sample and Hold1/1 -> Sum1/2
  Clock1/1 -> Sample and Hold1/1
  Constant20/1 -> Switch13/3
  Sum1/1 -> Switch13/1
  Constant21/1 -> Switch15/1
  Constant3/1 -> Switch15/3
  Clock3/1 -> Sum1/1
  Switch15/1 -> Sample and Hold2/Trigger, Switch14/2, Switch1/2
  Trigger/1 -> Switch13/2, Sample and Hold1/Trigger
  Switch2/1 -> Out/1, [recover_en]

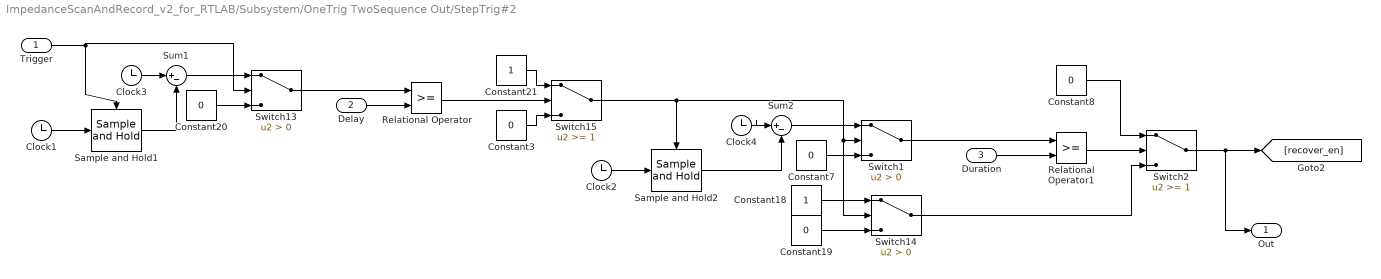
== system ImpedanceScanAndRecord_v2_for_RTLAB/Subsystem/OneTrig TwoSequence Out/StepTrig#2 ==
  Trigger : Inport
  Delay : Inport  Port=2
  Duration : Inport  Port=3
  Clock{1..4} (4 alike) : Clock
      Clock3 settings: DisableCoverage=on
      Clock4 settings: DisableCoverage=on
  Constant18 : Constant
  Constant{3,7..8,19..20} (5 alike) : Constant  Value=0
  Constant21 : Constant
  Relational Operator : RelationalOperator  OutDataTypeStr=boolean  RndMeth=Nearest
  Relational Operator1 : RelationalOperator  OutDataTypeStr=boolean  RndMeth=Nearest
  Sample and Hold1 : dspsigops/Sample and Hold  trig=Rising edge  initCond=0  latchinput=off
  Sample and Hold2 : dspsigops/Sample and Hold  trig=Rising edge  initCond=0  latchinput=off
  Sum1 : Sum  DisableCoverage=on  Inputs=|+-  InputSameDT=on  SaturateOnIntegerOverflow=on  OutDataTypeStr=Inherit: Same as first input
  Sum2 : Sum  DisableCoverage=on  Inputs=|+-  InputSameDT=on  SaturateOnIntegerOverflow=on  OutDataTypeStr=Inherit: Same as first input
  Switch1 : Switch  Criteria=u2 > Threshold  SampleTime=var_myts
  Switch13 : Switch  Criteria=u2 > Threshold  SampleTime=var_myts
  Switch14 : Switch  Criteria=u2 > Threshold  SampleTime=var_myts
  Switch15 : Switch  Threshold=1  SampleTime=var_myts
  Switch2 : Switch  Threshold=1  SampleTime=var_myts
  Out : Outport
  wires:
  Switch2/1 -> [recover_en], Out/1
  Trigger/1 -> Sample and Hold1/Trigger, Switch13/2
  Switch15/1 -> Switch1/2, Switch14/2, Sample and Hold2/Trigger
  Clock3/1 -> Sum1/1
  Constant3/1 -> Switch15/3
  Constant21/1 -> Switch15/1
  Sum1/1 -> Switch13/1
  Constant20/1 -> Switch13/3
  Clock1/1 -> Sample and Hold1/1
  Sample and Hold1/1 -> Sum1/2
  Constant19/1 -> Switch14/3
  Switch14/1 -> Switch2/3
  Constant7/1 -> Switch1/3
  Clock4/1 -> Sum2/1
  Constant8/1 -> Switch2/1
  Sample and Hold2/1 -> Sum2/2
  Constant18/1 -> Switch14/1
  Sum2/1 -> Switch1/1
  Clock2/1 -> Sample and Hold2/1
  Switch13/1 -> Relational Operator/1
  Delay/1 -> Relational Operator/2
  Relational Operator/1 -> Switch15/2
  Relational Operator1/1 -> Switch2/2
  Switch1/1 -> Relational Operator1/1
  Duration/1 -> Relational Operator1/2

== matlab function ImpedanceScanAndRecord_v2_for_RTLAB/Impedance Scan/MATLAB Function1 ==
  data: t input; duration input; y output; trig input
function y = fcn(t, duration, trig)

persistent trig_now trig_last t_start state_change
    if isempty(trig_now)
        trig_now = 0;
    end

    if isempty(trig_last)
        trig_last = 0;
    end
    
    if isempty(t_start)
        t_start = 0;
    end
    
    
    if isempty(state_change)
        state_change = 0;
    end

trig_now = trig;
if trig_now ~= trig_last
    state_change = 1;
    t_start = t;
end

if state_change == 1
    if t - t_start > duration
        state_change = 0;
    end
end

trig_last = trig_now;
y = state_change;

== matlab function ImpedanceScanAndRecord_v2_for_RTLAB/MATLAB Function ==
  data: t input; duration input; y output; trig input
function y = fcn(t, duration, trig)

persistent trig_now trig_last t_start state_change
    if isempty(trig_now)
        trig_now = 0;
    end

    if isempty(trig_last)
        trig_last = 0;
    end
    
    if isempty(t_start)
        t_start = 0;
    end
    
    
    if isempty(state_change)
        state_change = 0;
    end

trig_now = trig;
if trig_now ~= trig_last
    state_change = 1;
    t_start = t;
end

if state_change == 1
    if t - t_start > duration
        state_change = 0;
    end
end

trig_last = trig_now;
y = state_change;

== matlab function ImpedanceScanAndRecord_v2_for_RTLAB/Impedance Scan/MATLAB Function ==
  data: Percent output; Enable input; InjectLen input; RecordLen input; StableLen input; InjectEn output; RecordEn output; StableEn output
function [Percent, InjectEn, RecordEn, StableEn] = fcn(Enable, InjectLen, RecordLen, StableLen)

persistent cnt_idx;
if isempty(cnt_idx)
    cnt_idx = 0;
    InjectEn = 0;
    RecordEn = 0;
    StableEn = 0;
else
    if Enable == 1
        if cnt_idx > 0 && cnt_idx <= (InjectLen-RecordLen)
            InjectEn = 1;
            RecordEn = 0;
            StableEn = 0;
        elseif cnt_idx > (InjectLen-RecordLen) && cnt_idx <= InjectLen
            InjectEn = 1;
            RecordEn = 1;
            StableEn = 0;
        elseif cnt_idx > InjectLen && cnt_idx <= (InjectLen + StableLen)
            InjectEn = 0;
            RecordEn = 0;
            StableEn = 1;
        else
            InjectEn = 0;
            RecordEn = 0;
            StableEn = 0;
        end
        cnt_idx = cnt_idx + 1;
    else
        cnt_idx = 0;
        InjectEn = 0;
        RecordEn = 0;
        StableEn = 0;
    end
end

Percent = cnt_idx;

== matlab function ImpedanceScanAndRecord_v2_for_RTLAB/Edge-trigger event ==
  data: t input; duration input; y output; trig input; trig_mode input
function y = fcn(t, duration, trig, trig_mode)
% trig_mode: 1 for rising-edge trigger, 2 for falling-edge trigger;
% static var declaration
persistent trig_now trig_last t_start state_change rise_trig fall_trig
    if isempty(trig_now)
        trig_now = 0;
    end

    if isempty(trig_last)
        trig_last = 0;
    end
    
    if isempty(t_start)
        t_start = 0;
    end
    
    if isempty(rise_trig)
        rise_trig = 0;
    end
    
    if isempty(fall_trig)
        fall_trig = 0;
    end
    
    if isempty(trig_mode)
        trig_mode = 0;
    end
    
    if isempty(state_change)
        state_change = 0;
    end

% Event catch depend on trig_mode
trig_now = trig;
if trig_now ~= trig_last
    if trig_now > trig_last
        if trig_mode == 1
            rise_trig = 1;
        end
    elseif trig_now < trig_last
        if trig_mode == 2
            fall_trig = 1;
        end
    end
    state_change = 1;
    t_start = t;
end

if state_change == 1
    if t - t_start > duration  % Some criteria
        % Your code here ...
        if trig_mode == 1
            rise_trig = 0;
        elseif trig_mode == 2
            fall_trig = 0;
        else
            state_change = 0;
        end  
    end
end

trig_last = trig_now;
if trig_mode == 1
    y = rise_trig;
elseif trig_mode == 2
    y = fall_trig;
else
    y = state_change;
end

== matlab function ImpedanceScanAndRecord_v2_for_RTLAB/Edge-trigger counter ==
  data: cnt_begin input; cnt_step input; cnt_end input; trig input; trig_mode input; cnt_out output
function cnt_out = fcn(cnt_begin, cnt_step, cnt_end, trig, trig_mode)
% trig_mode: 1 for rising-edge trigger, 2 for falling-edge trigger;
% static var declaration
persistent trig_now trig_last  rise_trig fall_trig cnt
    if isempty(trig_now)
        trig_now = 0;
    end

    if isempty(trig_last)
        trig_last = 0;
    end
    
    if isempty(rise_trig)
        rise_trig = 0;
    end
    
    if isempty(fall_trig)
        fall_trig = 0;
    end
    
    if isempty(trig_mode)
        trig_mode = 0;
    end
    
    if isempty(cnt)
        cnt = cnt_begin;
    end

% Event catch depend on trig_mode
trig_now = trig;
if trig_now ~= trig_last
    if trig_now > trig_last
        if trig_mode == 1
            rise_trig = 1;
            % Your code here...
        end
    elseif trig_now < trig_last
        if trig_mode == 2
            fall_trig = 1;
            % Your code here...
            cnt = cnt + cnt_step;
            if cnt > cnt_end
                cnt = cnt_begin;
            end
        end
    end
end

trig_last = trig_now;

cnt_out = cnt

== matlab function ImpedanceScanAndRecord_v2_for_RTLAB/MATLAB Function1 ==
  data: t input; trig input; y output; duration input
function y = fcn(t, trig, duration)
%#codegen
persistent trig_now trig_last t_start state_change rise_trig fall_trig
    if isempty(trig_now)
        trig_now = 0;
    end
    if isempty(trig_last)
        trig_last = 0;
    end
    if isempty(t_start)
        t_start = 0;
    end
    if isempty(state_change)
        state_change = 0;
    end
    if isempty(rise_trig)
        rise_trig = 0;
    end
    
    if isempty(fall_trig)
        fall_trig = 0;
    end
    
    
trig_now = trig;
if trig_now ~= trig_last
    if trig_now > trig_last
        rise_trig = 1;
    elseif trig_now < trig_last
        fall_trig = 1;
    end
    state_change = 1;
    t_start = t;
end

if state_change == 1
    if t - t_start > duration
        state_change = 0;
        rise_trig = 0;
        fall_trig = 0;
    end
end

trig_last = trig_now;
y = fall_trig;

== matlab function ImpedanceScanAndRecord_v2_for_RTLAB/Subsystem/Edge-trigger counter ==
  data: cnt_begin input; cnt_step input; cnt_end input; trig input; trig_mode input; cnt_out output
function cnt_out = fcn(cnt_begin, cnt_step, cnt_end, trig, trig_mode)
% trig_mode: 1 for rising-edge trigger, 2 for falling-edge trigger;
% static var declaration
persistent trig_now trig_last  rise_trig fall_trig cnt
    if isempty(trig_now)
        trig_now = 0;
    end

    if isempty(trig_last)
        trig_last = 0;
    end
    
    if isempty(rise_trig)
        rise_trig = 0;
    end
    
    if isempty(fall_trig)
        fall_trig = 0;
    end
    
    if isempty(trig_mode)
        trig_mode = 0;
    end
    
    if isempty(cnt)
        cnt = cnt_begin;
    end

% Event catch depend on trig_mode
trig_now = trig;
if trig_now ~= trig_last
    if trig_now > trig_last
        if trig_mode == 1
            rise_trig = 1;
            % Your code here...
        end
    elseif trig_now < trig_last
        if trig_mode == 2
            fall_trig = 1;
            % Your code here...
            cnt = cnt + cnt_step;
            if cnt > cnt_end
                cnt = cnt_begin;
            end
        end
    end
end

trig_last = trig_now;

cnt_out = cnt
